simulink model "zad1"  (R2023b)
settings: Solver=VariableStepAuto  StartTime=0.0  StopTime=80  RelTol=1e-3
settings Model: Creator=KMPKM  LastModifiedBy=KMPKM

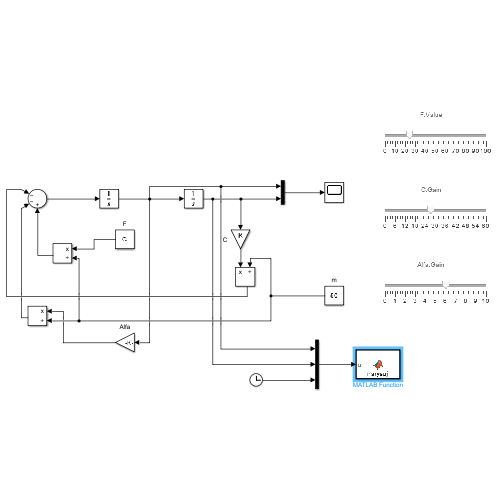
[thumbnail: Simulink's stored preview of the top-level diagram]
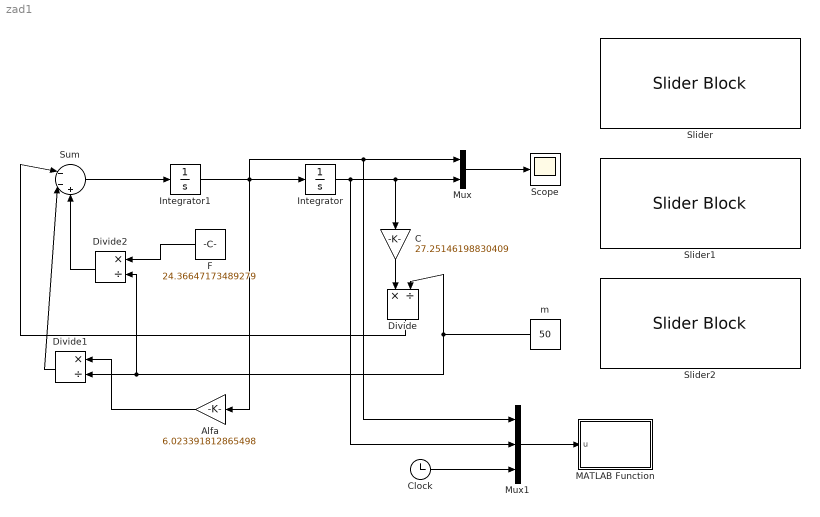
== system zad1 ==
  Alfa : Gain  Gain=6.023391812865498
  C : Gain  Gain=27.25146198830409
  Clock : Clock
  Divide : Product  Inputs=*/
  Divide1 : Product  Inputs=*/
  Divide2 : Product  Inputs=*/
  F : Constant  Value=24.36647173489279
  Integrator : Integrator
  Integrator1 : Integrator
  MATLAB Function : MATLAB Function  TreatAsAtomicUnit=on
  Mux : Mux  Inputs=2
  Mux1 : Mux  Inputs=3
  Scope : Scope
  Slider : SliderBlock
  Slider1 : SliderBlock  ScaleMax=60
  Slider2 : SliderBlock  ScaleMax=10  TickInterval=1
  Sum : Sum  Inputs=|--+
  m : Constant  Value=50
  wires:
  Sum/1 -> Integrator1/1
  Mux/1 -> Scope/1
  C/1 -> Divide/1
  m/1 -> Divide2/2, Divide1/2, Divide/2
  Alfa/1 -> Divide1/1
  Divide/1 -> Sum/1
  Divide1/1 -> Sum/2
  F/1 -> Divide2/1
  Divide2/1 -> Sum/3
  Integrator1/1 -> Alfa/1, Mux1/1, Mux/1, Integrator/1
  Integrator/1 -> Mux1/2, C/1, Mux/2
  Mux1/1 -> MATLAB Function/1(u)
  Clock/1 -> Mux1/3

== matlab function zad1/MATLAB Function ==
  data: u input
function narysuj(u)

x = u(1);
y = u(2);
t = u(3);


cla
figure
plot(x,y,'b', 'LineWidth',1.5)
hold on
plot(x,t, '--r')
grid
drawnow
